simulink model "simulink_model_parteB"  (R2023b)
settings: Solver=VariableStepAuto  StartTime=0.0  StopTime=100  RelTol=1e-3
libraries: fuzblock x1
settings Model: Creator=jbsantos  LastModifiedBy=jbsantos

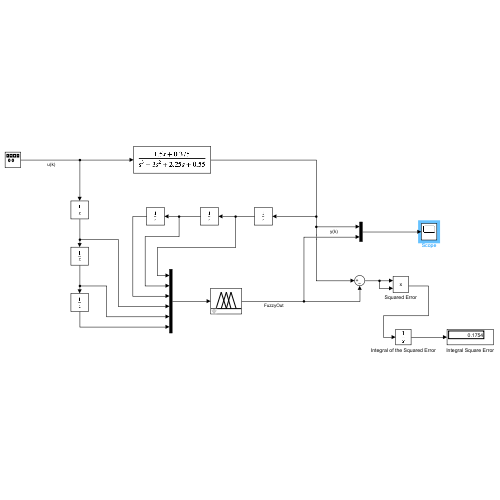
[thumbnail: Simulink's stored preview of the top-level diagram]
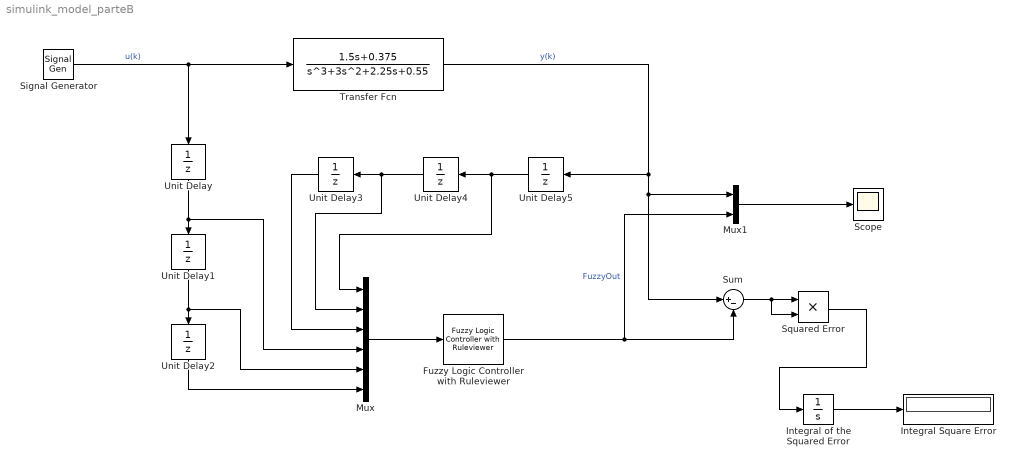
== system simulink_model_parteB ==
  Fuzzy Logic Controller with Ruleviewer : fuzblock/Fuzzy Logic  Controller  with Ruleviewer  fismatrix=fis_sc0  Ts=0.5
  Integral Square Error : Display
  Integral of the Squared Error : Integrator
  Mux : Mux  Inputs=6
  Mux1 : Mux  Inputs=2
  Scope : Scope
  Signal Generator : SignalGenerator  WaveForm=sawtooth  Frequency=0.1  Units=rad/sec
  Squared Error : Product
  Sum : Sum  Inputs=|+-
  Transfer Fcn : TransferFcn  Numerator=[1.5 0.375]  Denominator=[1 3 2.25 0.55]
  Unit Delay{,1..5} (6 alike) : UnitDelay  SampleTime=-1  HasFrameUpgradeWarning=on
  wires:
  Signal Generator/1 -> Unit Delay/1, Transfer Fcn/1  "u(k)"
  Transfer Fcn/1 -> Unit Delay5/1, Mux1/1, Sum/1  "y(k)"
  Unit Delay5/1 -> Unit Delay4/1, Mux/1
  Unit Delay4/1 -> Mux/2, Unit Delay3/1
  Unit Delay3/1 -> Mux/3
  Unit Delay/1 -> Mux/4, Unit Delay1/1
  Unit Delay1/1 -> Mux/5, Unit Delay2/1
  Unit Delay2/1 -> Mux/6
  Mux/1 -> Fuzzy Logic Controller with Ruleviewer/1
  Fuzzy Logic Controller with Ruleviewer/1 -> Sum/2, Mux1/2  "FuzzyOut"
  Mux1/1 -> Scope/1
  Sum/1 -> Squared Error/1, Squared Error/2
  Squared Error/1 -> Integral of the Squared Error/1
  Integral of the Squared Error/1 -> Integral Square Error/1
